simulink model "TP1_simu_IV1"  (R2020a)
settings: Solver=VariableStepAuto  StartTime=0.0  StopTime=50  RelTol=1e-3
undefined symbols (not defined in the file): h, kd, kp, L, r, tau
settings Model: Creator=ferrei177u  LastModifiedBy=deric
settings OptimizationCC: LifeSpan=inf
settings DebuggingCC: UnconnectedInputMsg=none  UnconnectedOutputMsg=none  UnconnectedLineMsg=none  ArithmeticOperatorsInVariantConditions=warning
settings SFSimCC: CustomCodeUndefinedFunction=UseInterfaceOnly
settings CodeAppCC: StateflowObjectComments=on

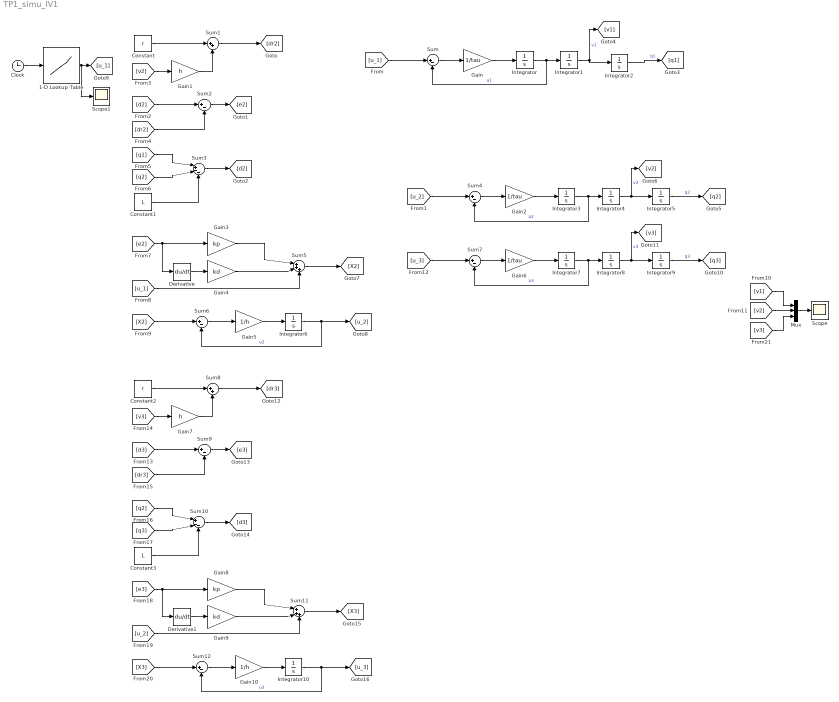
== system TP1_simu_IV1 ==
  1-D Lookup Table : Lookup_n-D  NumberOfTableDimensions=1  BreakpointsForDimension1=[0 1 4 10 13 14]  Table=tanh([0 0 -3 3 0 0])  InternalRulePriority=Speed  RndMeth=Simplest  InputSameDT=on
  Clock : Clock
  Constant : Constant  Value=r
  Constant1 : Constant  Value=L
  Constant2 : Constant  Value=r
  Constant3 : Constant  Value=L
  Derivative : Derivative
  Derivative1 : Derivative
  Gain : Gain  Gain=1/tau
  Gain1 : Gain  Gain=h
  Gain10 : Gain  Gain=1/h
  Gain2 : Gain  Gain=1/tau
  Gain3 : Gain  Gain=kp
  Gain4 : Gain  Gain=kd
  Gain5 : Gain  Gain=1/h
  Gain6 : Gain  Gain=1/tau
  Gain7 : Gain  Gain=h
  Gain8 : Gain  Gain=kp
  Gain9 : Gain  Gain=kd
  Integrator{,3,6..7,9..10} (6 alike) : Integrator
  Integrator1 : Integrator  InitialCondition=130
  Integrator2 : Integrator  InitialCondition=2*L+2*r+2*h*130
  Integrator4 : Integrator  InitialCondition=130
  Integrator5 : Integrator  InitialCondition=L+r+h*130
  Integrator8 : Integrator  InitialCondition=130
  Mux : Mux  Inputs=3
  Scope : Scope
  Scope1 : Scope
  Sum{,2,4,6..7,9,12} (7 alike) : Sum  Inputs=|+-
  Sum1 : Sum  Inputs=|++
  Sum10 : Sum  Inputs=|+--
  Sum11 : Sum  Inputs=|+++
  Sum3 : Sum  Inputs=|+--
  Sum5 : Sum  Inputs=|+++
  Sum8 : Sum  Inputs=|++
  wires:
  Gain/1 -> Integrator/1
  Sum/1 -> Gain/1
  [u_1] -> Sum/1
  Integrator/1 -> Integrator1/1, Sum/2  "a1"
  Constant/1 -> Sum1/1
  [v2] -> Gain1/1
  Sum1/1 -> [dr2]
  [d2] -> Sum2/1
  Sum2/1 -> [e2]
  [q1] -> Sum3/1
  [q2] -> Sum3/2
  Constant1/1 -> Sum3/3
  Sum3/1 -> [d2]
  Integrator1/1 -> [v1], Integrator2/1  "v1"
  Integrator2/1 -> [q1]  "q1"
  [u_2] -> Sum4/1
  Sum4/1 -> Gain2/1
  Integrator4/1 -> [v2], Integrator5/1  "v2"
  Integrator3/1 -> Integrator4/1, Sum4/2  "a2"
  Integrator5/1 -> [q2]  "q2"
  Gain2/1 -> Integrator3/1
  [e2] -> Derivative/1, Gain3/1
  Derivative/1 -> Gain4/1
  Gain3/1 -> Sum5/1
  Gain4/1 -> Sum5/2
  Sum5/1 -> [X2]
  [X2] -> Sum6/1
  Sum6/1 -> Gain5/1
  Gain5/1 -> Integrator6/1
  Integrator6/1 -> [u_2], Sum6/2  "u2"
  Gain1/1 -> Sum1/2
  [dr2] -> Sum2/2
  [v1] -> Mux/1
  [v2] -> Mux/2
  Mux/1 -> Scope/1
  Clock/1 -> 1-D Lookup Table/1
  1-D Lookup Table/1 -> Scope1/1, [u_1]
  Integrator8/1 -> [v3], Integrator9/1  "v3"
  Integrator7/1 -> Integrator8/1, Sum7/2  "a3"
  Sum7/1 -> Gain6/1
  [u_3] -> Sum7/1
  Gain6/1 -> Integrator7/1
  Integrator9/1 -> [q3]  "q3"
  Sum11/1 -> [X3]
  [dr3] -> Sum9/2
  [v3] -> Gain7/1
  Constant2/1 -> Sum8/1
  [q2] -> Sum10/1
  Sum8/1 -> [dr3]
  Sum10/1 -> [d3]
  Constant3/1 -> Sum10/3
  Gain8/1 -> Sum11/1
  Gain7/1 -> Sum8/2
  [d3] -> Sum9/1
  Integrator10/1 -> [u_3], Sum12/2  "u3"
  [X3] -> Sum12/1
  [e3] -> Derivative1/1, Gain8/1
  Derivative1/1 -> Gain9/1
  Sum12/1 -> Gain10/1
  [q3] -> Sum10/2
  Gain9/1 -> Sum11/2
  Sum9/1 -> [e3]
  Gain10/1 -> Integrator10/1
  [v3] -> Mux/3
  [u_1] -> Sum5/3
  [u_2] -> Sum11/3
